simulink model "pendulumSIM"  (R2016a)
settings: Solver=ode45  StartTime=0.0  StopTime=10.0  MaxStep=0.05  RelTol=1e-3
values from neighbouring files (symbols this model uses):
  g = 9.81    [ConstPendulum.m]    (also in VarPendulum.m)
  r = zeros(length(theta))    [Wrapper.m]    (also in body.m = 0.8)
undefined symbols (not defined in the file or in its folder): drdtheta, drdtheta_dot, theta_dot_initial, theta_initial
settings Model: Creator=richard.hill  LastModifiedBy=Arjun
settings DataIOCC: LimitDataPoints=on  SaveFormat=Array
settings DebuggingCC: UnderspecifiedInitializationDetection=Classic  MergeDetectMultiDrivingBlocksExec=none  SolverPrmCheckMsg=warning
settings HardwareCC: ProdBitPerPointer=32  ProdLargestAtomicFloat=None  ProdIntDivRoundTo=Undefined  ProdEndianess=Unspecified  ProdWordSize=32  ProdHWDeviceType=32-bit Generic
settings ModelReferenceCC: PropagateSignalLabelsOutOfModel=off
settings ConfigComp: CovModelRefEnable=Off

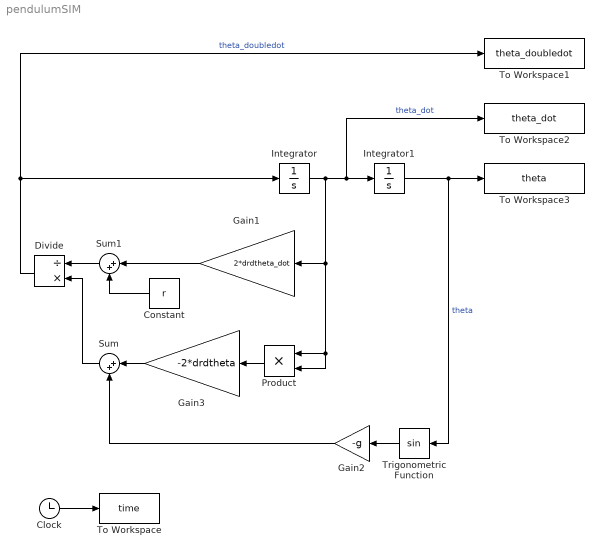
== system pendulumSIM ==
  Clock : Clock
  Constant : Constant  Value=r
  Divide : Product  Inputs=/*
  Gain1 : Gain  Gain=2*drdtheta_dot
  Gain2 : Gain  Gain=-g
  Gain3 : Gain  Gain=-2*drdtheta
  Integrator : Integrator  InitialCondition=theta_dot_initial
  Integrator1 : Integrator  InitialCondition=theta_initial
  Product : Product
  Sum : Sum  Inputs=|++
  Sum1 : Sum  Inputs=|++
  To Workspace : ToWorkspace  VariableName=time  SampleTime=-1
  To Workspace1 : ToWorkspace  VariableName=theta_doubledot  SampleTime=-1
  To Workspace2 : ToWorkspace  VariableName=theta_dot  SampleTime=-1
  To Workspace3 : ToWorkspace  VariableName=theta  SampleTime=-1
  Trigonometric Function : Trigonometry
  wires:
  Divide/1 -> To Workspace1/1, Integrator/1  "theta_doubledot"
  Integrator/1 -> Product/2, Product/1, Gain1/1, Integrator1/1, To Workspace2/1  "theta_dot"
  Integrator1/1 -> Trigonometric Function/1, To Workspace3/1  "theta"
  Trigonometric Function/1 -> Gain2/1
  Clock/1 -> To Workspace/1
  Product/1 -> Gain3/1
  Gain3/1 -> Sum/1
  Gain2/1 -> Sum/2
  Sum/1 -> Divide/2
  Gain1/1 -> Sum1/1
  Constant/1 -> Sum1/2
  Sum1/1 -> Divide/1
